simulink model "Machinesprj2main19a"  (R2020a)
settings: Solver=ode23  StartTime=0.0  StopTime=20  RelTol=1e-6
values from neighbouring files (symbols this model uses):
  f_abc = 60    [Machinesprj2.m]
  i_f = Vfd/Rf    (= 12000)    [Machinesprj2.m]
  ids = 0    [Machinesprj2.m]
  invL = inv(L)    [Machinesprj2.m]
  iqs = sqrt(7.9674e+03)    [Machinesprj2.m]
  J = 35.1e6    (= 35100000)    [Machinesprj2.m]
  JL = Jmatrix*L    [Machinesprj2.m]
  L = eye(7)    [Machinesprj2.m]
  P = 64    [Machinesprj2.m]
  R = eye(7)    [Machinesprj2.m]
  theta_e0 = theta_r0*P/2    (= 0)    [Machinesprj2.m]
  theta_r0 = 0    [Machinesprj2.m]
  Vfd = 6    [Machinesprj2.m]
  Vs_abc = 20e3*sqrt(2)/sqrt(3)    [Machinesprj2.m]
  wb = 112.5*2*pi/60    (= 11.780972451)    [Machinesprj2.m]
settings Model: Creator=15043  LastModifiedBy=venka
settings SFSimCC: CustomCodeUndefinedFunction=UseInterfaceOnly

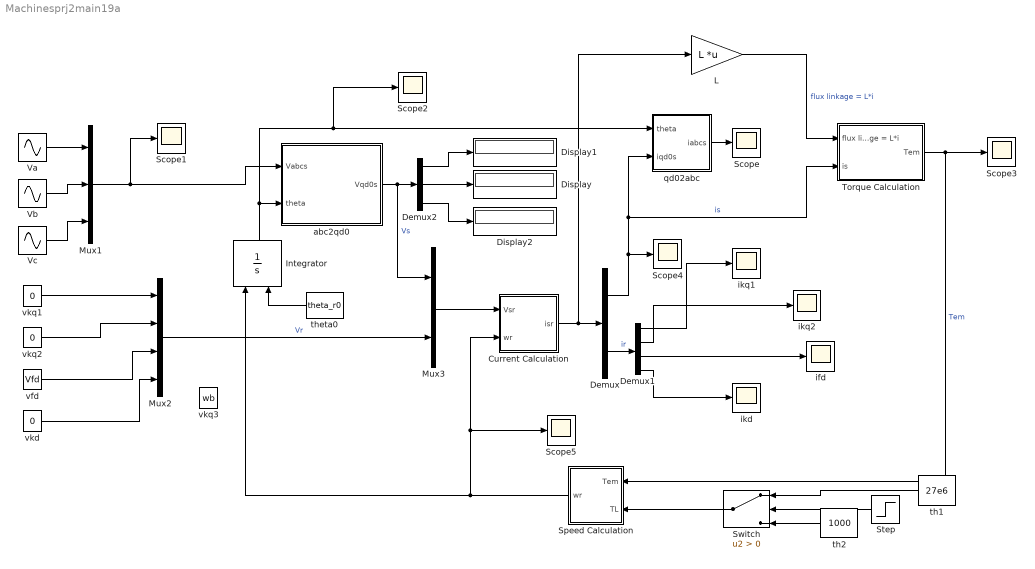
== system Machinesprj2main19a ==
  Current Calculation : Subsystem
  Demux : Demux  Outputs=[3 4]
  Demux1 : Demux
  Demux2 : Demux  Outputs=3
  Display : Display
  Display1 : Display
  Display2 : Display
  Integrator : Integrator  InitialConditionSource=external
  L : Gain  Gain=L  Multiplication=Matrix(K*u) (u vector)
  Mux1 : Mux  Inputs=3
  Mux2 : Mux
  Mux3 : Mux  Inputs=[3 4]
  Scope{,1..5} (6 alike) : Scope
  Speed Calculation : Subsystem
  Step : Step  Time=4  SampleTime=0
  Switch : Switch  Criteria=u2 > Threshold
  Torque Calculation : Subsystem
  Va : Sin  Amplitude=Vs_abc  Frequency=f_abc*2*pi  Phase=theta_e0+pi/2  SampleTime=0
  "Vb " : Sin  Amplitude=Vs_abc  Frequency=f_abc*2*pi  Phase=theta_e0-2*pi/3+pi/2  SampleTime=0
  Vc : Sin  Amplitude=Vs_abc  Frequency=f_abc*2*pi  Phase=theta_e0+2*pi/3+pi/2  SampleTime=0
  abc2qd0 : Subsystem
  ifd : Scope
  ikd : Scope
  ikq1 : Scope
  ikq2 : Scope
  qd02abc : Subsystem
  th1 : Constant  Value=27e6
  th2 : Constant  Value=1000
  theta0 : Constant  Value=theta_r0
  vfd : Constant  Value=Vfd
  vkd : Constant  Value=0
  vkq1 : Constant  Value=0
  vkq2 : Constant  Value=0
  vkq3 : Constant  Value=wb
  wires:
  Va/1 -> Mux1/1
  Mux1/1 -> Scope1/1, abc2qd0/1(Vabcs)
  vkq1/1 -> Mux2/1
  abc2qd0/1(Vqd0s) -> Demux2/1, Mux3/1  "Vs"
  Mux2/1 -> Mux3/2  "Vr"
  theta0/1 -> Integrator/2
  vkq2/1 -> Mux2/2
  vfd/1 -> Mux2/3
  vkd/1 -> Mux2/4
  Mux3/1 -> Current Calculation/1(Vsr)
  Current Calculation/1(isr) -> L/1, Demux/1
  Demux/2 -> Demux1/1  "ir"
  Integrator/1 -> abc2qd0/2("theta "), Scope2/1, qd02abc/1(theta)
  Demux/1 -> Scope4/1, qd02abc/2(iqd0s), Torque Calculation/2(is)  "is"
  qd02abc/1(iabcs) -> Scope/1
  Demux1/1 -> ikq1/1
  Demux1/2 -> ikq2/1
  Demux1/3 -> ifd/1
  Demux1/4 -> ikd/1
  L/1 -> Torque Calculation/1(flux linkage = L*i)  "flux linkage = L*i"
  Torque Calculation/1(Tem) -> Scope3/1, Speed Calculation/1(Tem)  "Tem"
  Switch/1 -> Speed Calculation/2(TL)
  Speed Calculation/1(wr) -> Integrator/1, Current Calculation/2(wr), Scope5/1
  "Vb "/1 -> Mux1/2
  Vc/1 -> Mux1/3
  Demux2/2 -> Display/1
  Demux2/1 -> Display1/1
  Demux2/3 -> Display2/1
  th1/1 -> Switch/1
  th2/1 -> Switch/3
  Step/1 -> Switch/2

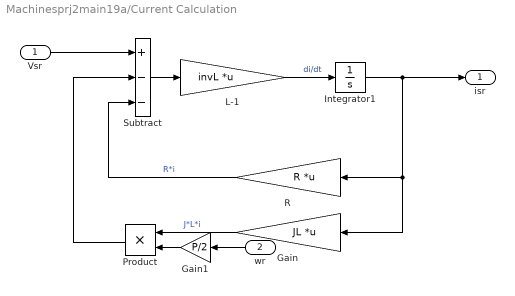
== system Machinesprj2main19a/Current Calculation ==
  Vsr : Inport
  wr : Inport  Port=2
  Gain : Gain  Gain=JL  Multiplication=Matrix(K*u) (u vector)
  Gain1 : Gain  Gain=P/2
  Integrator1 : Integrator  InitialCondition=[iqs;ids;0;0;0;i_f;0]
  L-1 : Gain  Gain=invL  Multiplication=Matrix(K*u) (u vector)
  Product : Product
  R : Gain  Gain=R  Multiplication=Matrix(K*u) (u vector)
  Subtract : Sum  Inputs=+--
  isr : Outport
  wires:
  Product/1 -> Subtract/2
  Gain/1 -> Product/1  "J*L*i"
  Subtract/1 -> L-1/1
  R/1 -> Subtract/3  "R*i"
  Vsr/1 -> Subtract/1
  Gain1/1 -> Product/2
  wr/1 -> Gain1/1
  L-1/1 -> Integrator1/1  "di/dt"
  Integrator1/1 -> Gain/1, R/1, isr/1

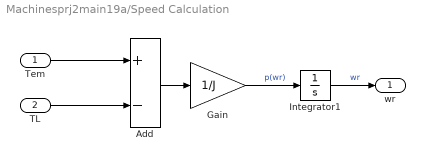
== system Machinesprj2main19a/Speed Calculation ==
  Tem : Inport
  TL : Inport  Port=2
  Add : Sum  Inputs=+-
  Gain : Gain  Gain=1/J
  Integrator1 : Integrator  InitialCondition=wb
  wr : Outport
  wires:
  Add/1 -> Gain/1
  TL/1 -> Add/2
  Gain/1 -> Integrator1/1  "p(wr)"
  Tem/1 -> Add/1
  Integrator1/1 -> wr/1  "wr"

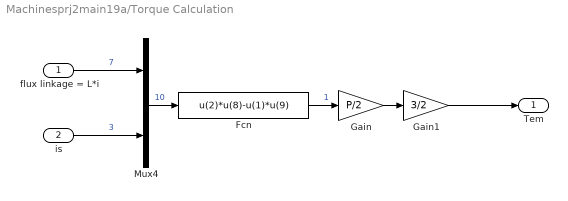
== system Machinesprj2main19a/Torque Calculation ==
  flux linkage = L*i : Inport
  is : Inport  Port=2
  Fcn : Fcn  Expr=u(2)*u(8)-u(1)*u(9)
  Gain : Gain  Gain=P/2
  Gain1 : Gain  Gain=3/2
  Mux4 : Mux  Inputs=[7 3]
  Tem : Outport
  wires:
  Gain1/1 -> Tem/1
  Gain/1 -> Gain1/1
  Mux4/1 -> Fcn/1  "10"
  flux linkage = L*i/1 -> Mux4/1  "7"
  Fcn/1 -> Gain/1  "1"
  is/1 -> Mux4/2  "3"

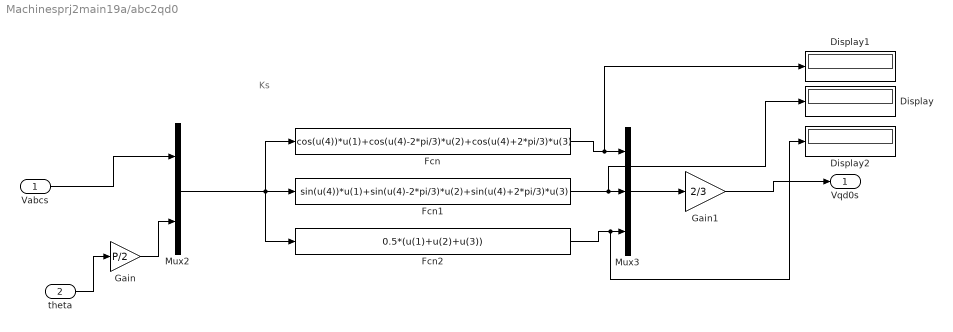
== system Machinesprj2main19a/abc2qd0 ==
  note: Ks
  Vabcs : Inport
  "theta " : Inport  Port=2
  Display : Display
  Display1 : Display
  Display2 : Display
  Fcn : Fcn  Expr=cos(u(4))*u(1)+cos(u(4)-2*pi/3)*u(2)+cos(u(4)+2*pi/3)*u(3)
  Fcn1 : Fcn  Expr=sin(u(4))*u(1)+sin(u(4)-2*pi/3)*u(2)+sin(u(4)+2*pi/3)*u(3)
  Fcn2 : Fcn  Expr=0.5*(u(1)+u(2)+u(3))
  Gain : Gain  Gain=P/2
  Gain1 : Gain  Gain=2/3
  Mux2 : Mux  Inputs=[3 1]
  Mux3 : Mux  Inputs=3
  Vqd0s : Outport
  wires:
  Fcn/1 -> Display1/1, Mux3/1
  Fcn1/1 -> Display/1, Mux3/2
  Mux2/1 -> Fcn2/1, Fcn1/1, Fcn/1
  Fcn2/1 -> Display2/1, Mux3/3
  Mux3/1 -> Gain1/1
  Gain1/1 -> Vqd0s/1
  "theta "/1 -> Gain/1
  Gain/1 -> Mux2/2
  Vabcs/1 -> Mux2/1

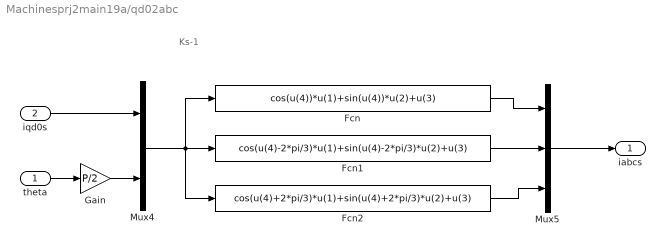
== system Machinesprj2main19a/qd02abc ==
  note: Ks-1
  theta : Inport
  iqd0s : Inport  Port=2
  Fcn : Fcn  Expr=cos(u(4))*u(1)+sin(u(4))*u(2)+u(3)
  Fcn1 : Fcn  Expr=cos(u(4)-2*pi/3)*u(1)+sin(u(4)-2*pi/3)*u(2)+u(3)
  Fcn2 : Fcn  Expr=cos(u(4)+2*pi/3)*u(1)+sin(u(4)+2*pi/3)*u(2)+u(3)
  Gain : Gain  Gain=P/2
  Mux4 : Mux  Inputs=[3 1]
  Mux5 : Mux  Inputs=3
  iabcs : Outport
  wires:
  iqd0s/1 -> Mux4/1
  Fcn/1 -> Mux5/1
  Mux4/1 -> Fcn2/1, Fcn1/1, Fcn/1
  Mux5/1 -> iabcs/1
  Fcn1/1 -> Mux5/2
  Fcn2/1 -> Mux5/3
  theta/1 -> Gain/1
  Gain/1 -> Mux4/2
